simulink model "Simulation_6DOFTesting01"  (R2024a)
settings: Solver=ode4  StartTime=initial_time  StopTime=final_time  FixedStep=timestep  RelTol=1e-3
values from neighbouring files (symbols this model uses):
  aEarth = 0    [CodeTesting_6DOF.m]    (also in Constants_6DOF.m = 6378137; Constants_6DOFTesting.m = 6378137)
  alphaArray = [-30, -25, -20, -15, -10, -5, 0, 5, 10, 15, 20, 25, 30]    [CodeTesting_6DOF.m]    (also in Constants_6DOF.m; Constants_6DOFTesting.m)
  altitudeArray = [0, 1000, 2000, 3000, 4000, 5000, 6000, 7000, 8000, 9000, 10000, 15000, 20000,      25000, 30000, 35000, 40000, 45000, 50000, 55000, 60000]    [CodeTesting_6DOF.m]    (also in Constants_6DOF.m; Constants_6DOFTesting.m)
  bEarth = 0    [CodeTesting_6DOF.m]    (also in Constants_6DOF.m = 6356752.3; Constants_6DOFTesting.m = 6356752.3)
  cD_3DArray = zeros(numAoAs, numMachs, numAltitudes)    [CodeTesting_6DOF.m]    (also in Constants_6DOF.m; Constants_6DOFTesting.m)
  cL_3DArray = zeros(numAoAs, numMachs, numAltitudes)    [CodeTesting_6DOF.m]    (also in Constants_6DOF.m; Constants_6DOFTesting.m)
  densityList = rhoList    [CodeTesting_6DOF.m]    (also in Constants_6DOF.m = usAtmosphere.x_; Constants_6DOFTesting.m = usAtmosphere.x_)
  height0 = 0    [Constants_6DOF.m]    (also in Constants_6DOFTesting.m = 5000)
  heightsList = usAtmosphere.Z    [CodeTesting_6DOF.m]    (also in Constants_6DOF.m; Constants_6DOFTesting.m)
  inertialPitch0 = deg2rad(inertialPitch0)    [Constants_6DOFTesting.m]
  inertialRoll0 = deg2rad(inertialRoll0)    [Constants_6DOFTesting.m]
  inertialYaw0 = deg2rad(inertialYaw0)    [Constants_6DOFTesting.m]
  Ixx = 10    [CodeTesting_6DOF.m]    (also in Constants_6DOF.m; Constants_6DOFTesting.m = 4.88094462)
  Ixz = 10    [CodeTesting_6DOF.m]    (also in Constants_6DOF.m = 1; Constants_6DOFTesting.m = 4.88094462)
  Iyy = 10    [CodeTesting_6DOF.m]    (also in Constants_6DOF.m; Constants_6DOFTesting.m = 4.88094462)
  Izz = 10    [CodeTesting_6DOF.m]    (also in Constants_6DOF.m; Constants_6DOFTesting.m = 4.88094462)
  latitude0 = pi/4    (= 0.785398163397)    [CodeTesting_6DOF.m]    (also in Constants_6DOF.m = deg2rad(latitude0); Constants_6DOFTesting.m = deg2rad(latitude0))
  longitude0 = pi/4    (= 0.785398163397)    [CodeTesting_6DOF.m]    (also in Constants_6DOF.m = deg2rad(longitude0); Constants_6DOFTesting.m = deg2rad(longitude0))
  m0 = 10    [CodeTesting_6DOF.m]    (also in Constants_6DOF.m = 50; Constants_6DOFTesting.m = 14.5939029)
  machArray = [0.5, 1.0, 1.5, 2.0, 2.5, 3.0, 3.5, 4.0, 4.5, 5.0, 5.5, 6.0, 6.5, 7.0, 7.5, 8.0,      8.5, 9.0, 9.5, 10.0]    [CodeTesting_6DOF.m]    (also in Constants_6DOF.m; Constants_6DOFTesting.m)
  omegaEarth = omega_earth    (= 7.2921159e-05)    [CodeTesting_6DOF.m]    (also in Constants_6DOF.m; Constants_6DOFTesting.m)
  p0Body = deg2rad(p0Body)    [Constants_6DOFTesting.m]
  phiBody0 = deg2rad(phiBody0)    [Constants_6DOFTesting.m]
  pitchCharacteristicLength = 0.0    (= 0)    [Constants_6DOFTesting.m]
  psiBody0 = deg2rad(psiBody0)    [Constants_6DOFTesting.m]
  q0Body = deg2rad(q0Body)    [Constants_6DOFTesting.m]
  r0Body = deg2rad(r0Body)    [Constants_6DOFTesting.m]
  rEarth = r_earth    (= 6371008.8)    [CodeTesting_6DOF.m]    (also in Constants_6DOF.m; Constants_6DOFTesting.m)
  rollCharacteristicLength = 0.0    (= 0)    [Constants_6DOFTesting.m]
  temperatureList = usAtmosphere.T    [CodeTesting_6DOF.m]    (also in Constants_6DOF.m; Constants_6DOFTesting.m)
  thetaBody0 = deg2rad(thetaBody0)    [Constants_6DOFTesting.m]
  u0Body = 304.8    [Constants_6DOFTesting.m]
  v0Body = 0    [Constants_6DOFTesting.m]
  w0Body = -1 * w0Body    (= 0)    [Constants_6DOFTesting.m]
  wingArea = 0    [CodeTesting_6DOF.m]    (also in Constants_6DOF.m = 50; Constants_6DOFTesting.m = 0.09290304)
  yawCharacteristicLength = 0.0    (= 0)    [Constants_6DOFTesting.m]
undefined symbols (not defined in the file or in its folder): inertialX0, inertialY0, inertialZ0
libraries: simulink_extras x28
(part 2 of 2)

== matlab function Simulation_6DOFTesting01/Coordinate Transformations/ecef2ned ==
  data: positionECEF input; y output; latitude input; longitude input
function y = fcn(positionECEF, latitude, longitude)

rotationMatrix = [-sin(latitude) * cos(longitude) -sin(latitude) * sin(longitude) cos(latitude); -sin(longitude) cos(longitude) 0; -cos(latitude) * cos(longitude) -cos(latitude) * sin(longitude) sin(latitude)];

nedPosition = rotationMatrix * positionECEF;

y = nedPosition;

== matlab function Simulation_6DOFTesting01/Control Surfaces/bankAngle ==
  data: t input; y output
function y = fcn(t)

bankAngle = 0;

y = bankAngle;

== matlab function Simulation_6DOFTesting01/Forces, Moments & their Coefficients/rollCoeff ==
  data: rollSurfaceDeflection input; y output
function y = fcn(rollSurfaceDeflection)

staticRollCoeff = rollSurfaceDeflection;
dynamicRollCoeff = 0.0;

rollCoeff = staticRollCoeff + dynamicRollCoeff;

y = rollCoeff;

== matlab function Simulation_6DOFTesting01/Forces, Moments & their Coefficients/pitchCoeff ==
  data: pitchSurfaceDeflection input; y output
function y = fcn(pitchSurfaceDeflection)

staticPitchCoeff = pitchSurfaceDeflection;
dynamicPitchCoeff = 0.0;

pitchCoeff = staticPitchCoeff + dynamicPitchCoeff;

y = pitchCoeff;

== matlab function Simulation_6DOFTesting01/Forces, Moments & their Coefficients/yawCoeff ==
  data: yawSurfaceDeflection input; y output
function y = fcn(yawSurfaceDeflection)

staticYawCoeff = yawSurfaceDeflection;
dynamicYawCoeff = 0.0;

yawCoeff = staticYawCoeff + dynamicYawCoeff;

y = yawCoeff;

== matlab function Simulation_6DOFTesting01/Constants & Aircraft Parameters/thrustBurnRate ==
  data: t input; y output
function y = fcn(t)

thrustBurnRate = 0;

y = thrustBurnRate;

== matlab function Simulation_6DOFTesting01/Forces, Moments & their Coefficients/Fx ==
  data: thrustX input; y output; gravityX input; dragX input; coriolisX input
function y = fcn(thrustX, gravityX, dragX, coriolisX)

xForce = thrustX + gravityX + coriolisX - dragX;

y = xForce;

== matlab function Simulation_6DOFTesting01/Forces, Moments & their Coefficients/Fy ==
  data: thrustY input; y output; gravityY input; coriolisY input
function y = fcn(thrustY, gravityY, coriolisY)

yForce = thrustY + gravityY + coriolisY;

y = yForce;

== matlab function Simulation_6DOFTesting01/Forces, Moments & their Coefficients/Fz ==
  data: thrustZ input; y output; gravityZ input; liftZ input; coriolisZ input
function y = fcn(thrustZ, gravityZ, liftZ, coriolisZ)

zForce = thrustZ + gravityZ + coriolisZ - liftZ;

y = zForce;

== matlab function Simulation_6DOFTesting01/Forces, Moments & their Coefficients/MATLAB Function ==
  data: thrustX input; y output; thrustY input; thrustZ input
function y = fcn(thrustX, thrustY, thrustZ)

thrustMagnitude = sqrt(thrustX^2 + thrustY^2 + thrustZ^2);

y = thrustMagnitude;

== matlab function Simulation_6DOFTesting01/Coordinate Transformations/Subsystem/velocity ==
  data: u input; y output; v input; w input
function y = fcn(u, v, w)

velocity = sqrt(u^2 + v^2 + w^2);

y = velocity;

== matlab function Simulation_6DOFTesting01/Forces, Moments & their Coefficients/MATLAB Function1 ==
  data: forceVector input; y output; AoA input; sideslip input
function y = fcn(forceVector, AoA, sideslip)

rotationMatrix = [cos(AoA) * cos(sideslip) -cos(AoA) * sin(sideslip) -sin(AoA); sin(sideslip) cos(sideslip) 0; sin(AoA) * cos(sideslip) -sin(AoA) * sin(sideslip) cos(AoA)];

rotatedForceVector = rotationMatrix * forceVector;

y = rotatedForceVector;

== matlab function Simulation_6DOFTesting01/Forces, Moments & their Coefficients/MATLAB Function2 ==
  data: m input; g input; psi input; theta input; phi input; AoA input; y output; sideslip input
function y = fcn(m, g, psi, theta, phi, AoA, sideslip)

inertialGravity = [0; 0; m * g];

x0 = cos(psi);
x1 = cos(theta);
x2 = sin(psi);
x3 = sin(theta);
x4 = cos(phi);
x5 = x2*x4;
x6 = sin(phi);
x7 = x0*x6;
x8 = x0*x4;
x9 = x2*x6;

rotationMatrixBI = [x0 * x1 x3 * x7 - x5 x3 * x8 + x9; x1 * x2 x3 * x9 + x8 x3 * x5 - x7; -x3 x1 * x6 x1 * x4];

rotationBI = inv(rotationMatrixBI);
rotationWB = [cos(AoA) * cos(sideslip) -cos(AoA) * sin(sideslip) -sin(AoA); sin(sideslip) cos(sideslip) 0; sin(AoA) * cos(sideslip) -sin(AoA) * sin(sideslip) cos(AoA)];

bodyGravity = rotationBI * inertialGravity;
windGravity = rotationWB * bodyGravity;

y = windGravity;

== matlab function Simulation_6DOFTesting01/Equations of Motion/Subsystem2/MATLAB Function1 ==
  data: r input; y output; q input; phi input
function y = fcn(r, q, phi)

y = q * cos(phi) - r * sin(phi);

== matlab function Simulation_6DOFTesting01/Equations of Motion/Subsystem2/MATLAB Function2 ==
  data: r input; y output; q input; phi input; theta input
function y = fcn(r, q, phi, theta)

y = q * sin(phi) * sec(theta) + r * cos(phi) * sec(theta);

== matlab function Simulation_6DOFTesting01/Control Surfaces/sideslipAngle ==
  data: t input; y output
function y = fcn(t)

sideslipAngle = 0;

y = sideslipAngle;

== matlab function Simulation_6DOFTesting01/Equations of Motion/Subsystem2/MATLAB Function3 ==
  data: omegaEarth input; y output; latitude input; longitude input; positionNED input
function y = fcn(omegaEarth, latitude, longitude, positionNED)

omegaEarth = [0; 0; omegaEarth];

lat = latitude;
long = longitude;

row1 = [-cos(long) * sin(lat) -sin(long) -cos(lat) * cos(long)];
row2 = [-sin(lat) * sin(long) cos(long) -cos(lat) * sin(long)];
row3 = [cos(lat) 0 -sin(lat)];

rotationMatrix = inv([row1; row2; row3]);
velocityNEDFrame = rotationMatrix * omegaEarth;
positionNED = positionNED;

velNEDX = velocityNEDFrame(1);
velNEDY = velocityNEDFrame(2);
velNEDZ = velocityNEDFrame(3);

posNEDX = positionNED(1);
posNEDY = positionNED(2);
posNEDZ = positionNED(3);

velRotEarthX = velNEDY * posNEDZ - velNEDZ * posNEDY;
velRotEarthY = velNEDZ * posNEDX - velNEDX * posNEDZ;
velRotEarthZ = velNEDX * posNEDY - velNEDY * posNEDX;

velocityRotatingEarth = [velRotEarthX; velRotEarthY; velRotEarthZ];

y = velocityRotatingEarth;

== matlab function Simulation_6DOFTesting01/Equations of Motion/Subsystem2/MATLAB Function4 ==
  data: velocityRotatingEarth input; y output
function y = fcn(velocityRotatingEarth)

magnitudeRotatingEarth = norm(velocityRotatingEarth);

y = magnitudeRotatingEarth;

== matlab function Simulation_6DOFTesting01/Coordinate Transformations/MATLAB Function ==
  data: positionNED input; y output; latitude input; longitude input
function y = fcn(positionNED, latitude, longitude)

rotationY = roty(pi/2 + latitude);
rotationZ = rotz(-1 * longitude);

rotationMatrix = rotationZ * rotationY;

cartesianECEF = rotationMatrix * positionNED;

y = cartesianECEF;

== matlab function Simulation_6DOFTesting01/Coordinate Transformations/Polar ECEF - lat, long, height/MATLAB Function ==
  data: a input; y output; b input; xECEF input; yECEF input; latitude input; height0 input
function y = fcn(a, b, xECEF, yECEF, latitude, height0)

e = sqrt(1 - b^2/a^2);
p = sqrt(xECEF^2 + yECEF^2);

N = a / sqrt(1 - e^2 * sin(latitude)^2);
alt = p / cos(latitude) - (N + height0);


y = alt;

== matlab function Simulation_6DOFTesting01/Forces, Moments & their Coefficients/Coriolis Force ==
  data: m input; y output; omegaEarth input; latitude input; longitude input; vNEDX input; vNEDY input; vNEDZ input
function y = fcn(m, omegaEarth, latitude, longitude, vNEDX, vNEDY, vNEDZ)

lat = latitude;
long = longitude;

row1 = [-cos(long) * sin(lat) -sin(long) -cos(lat) * cos(long)];
row2 = [-sin(lat) * sin(long) cos(long) -cos(lat) * sin(long)];
row3 = [cos(lat) 0 -sin(lat)];

rotationMatrix = inv([row1; row2; row3]);
omegaNED = rotationMatrix * [0; 0; omegaEarth];

omegNEDX = omegaNED(1);
omegNEDY = omegaNED(2);
omegNEDZ = omegaNED(3);

coriolisX = -2 * m * (omegNEDY * vNEDZ - omegNEDZ * vNEDY);
coriolisY = -2 * m * (omegNEDZ * vNEDX - omegNEDX * vNEDZ);
coriolisZ = -2 * m * (omegNEDX * vNEDY - omegNEDY * vNEDX);

coriolisX = 0;
coriolisY = 0;
coriolisZ = 0;

coriolisForce = [coriolisX; coriolisY; coriolisZ];

y = coriolisForce;

== matlab function Simulation_6DOFTesting01/Control Surfaces/AoA ==
  data: t input; y output
function y = fcn(t)

AoA = 0;

y = AoA;

== matlab function Simulation_6DOFTesting01/Equations of Motion/Subsystem1/MATLAB Function2 ==
  data: angleVector input; y output; phi input; theta input; psi input
function y = fcn(angleVector, phi, theta, psi)

x0 = cos(psi);
x1 = cos(theta);
x2 = sin(psi);
x3 = sin(theta);
x4 = cos(phi);
x5 = x2*x4;
x6 = sin(phi);
x7 = x0*x6;
x8 = x0*x4;
x9 = x2*x6;

rotationMatrixIB = [x0 * x1 x3 * x7 - x5 x3 * x8 + x9; x1 * x2 x3 * x9 + x8 x3 * x5 - x7; -x3 x1 * x6 x1 * x4];

angleVectorNED = rotationMatrixIB * angleVector;

y = angleVectorNED;

== matlab function Simulation_6DOFTesting01/Coordinate Transformations/Cartesian ECEF - x, y, z/MATLAB Function4 ==
  data: positionECEF input; y output
function y = fcn(positionECEF)

rEarth = 6371.0088 * 10^3;

height = norm(positionECEF) - rEarth;

y = height;

== matlab function Simulation_6DOFTesting01/Equations of Motion/Subsystem1/MATLAB Function3 ==
  data: psi input; y output; theta input; phi input
function y = fcn(psi, theta, phi)

initialAngleVector = [phi; theta; psi];

x0 = cos(psi);
x1 = cos(theta);
x2 = sin(psi);
x3 = sin(theta);
x4 = cos(phi);
x5 = x2*x4;
x6 = sin(phi);
x7 = x0*x6;
x8 = x0*x4;
x9 = x2*x6;

rotationMatrixIB = [x0 * x1 x3 * x7 - x5 x3 * x8 + x9; x1 * x2 x3 * x9 + x8 x3 * x5 - x7; -x3 x1 * x6 x1 * x4];

eulerAngles = rotationMatrixIB * initialAngleVector;

y = eulerAngles;

== matlab function Simulation_6DOFTesting01/Coordinate Transformations/Cartesian ECEF - x, y, z/MATLAB Function ==
  data: u input; y output
function y = fcn(u)

y = norm(u);

== matlab function Simulation_6DOFTesting01/Coordinate Transformations/Polar ECEF - lat, long, height/MATLAB Function4 ==
  data: u input; y output
function y = fcn(u)

y = norm(u);

== matlab function Simulation_6DOFTesting01/Coordinate Transformations/Polar ECEF - lat, long, height/MATLAB Function5 ==
  data: latitude input; longitude input; positionNED input; y output; latitude0 input; longitude0 input; height0 input; a input; b input; t input
function y = fcn( latitude, longitude, positionNED, latitude0, longitude0, height0, a, b, t)

rEarth = 6371.0088 * 10^3; 

long = longitude;
lat = latitude;

row1 = [-cos(long) * sin(lat) -sin(long) -cos(lat) * cos(long)];
row2 = [-sin(lat) * sin(long) cos(long) -cos(lat) * sin(long)];
row3 = [cos(lat) 0 -sin(lat)];

rotationMatrix = [row1; row2; row3];

positionNED(3) = positionNED(3);

e = sqrt(1 - b^2/a^2);
N = a * (1 - e^2 * sin(latitude0)^2)^(-1/2);

initialECEFX = (height0 + N) * cos(latitude0) * cos(longitude0);
initialECEFY = (height0 + N) * cos(latitude0) * sin(longitude0);
initialECEFZ = (height0 + N * (1 - e^2)) * sin(latitude0);

initialECEFPosition = [initialECEFX; initialECEFY; initialECEFZ];


positionECEF = rotationMatrix * positionNED + initialECEFPosition;

y = positionECEF;

== matlab function Simulation_6DOFTesting01/Coordinate Transformations/Polar ECEF - lat, long, height/MATLAB Function6 ==
  data: t input; y output; latitude0 input; xECEF input; yECEF input; zECEF input; a input; b input
function y = fcn(t, latitude0, xECEF, yECEF, zECEF, a, b)

e = sqrt(1 - b^2/a^2);
e2 = sqrt(a^2/b^2 - 1);
p = sqrt(xECEF^2 + yECEF^2);

theta = atan2(zECEF * a, p * b);
lat = atan2(zECEF + e2^2 * b * sin(theta)^3, p - e^2 * a * cos(theta)^3);

if t == 0
    latitude = latitude0;
else
    latitude = lat;
end

y = latitude;

== matlab function Simulation_6DOFTesting01/Control Surfaces/rollSurfaceDeflection ==
  data: t input; y output
function y = fcn(t)

rollSurfaceDeflection = 0.0;

y = rollSurfaceDeflection;

== matlab function Simulation_6DOFTesting01/Coordinate Transformations/Polar ECEF - lat, long, height/MATLAB Function7 ==
  data: t input; y output; longitude0 input; xECEF input; yECEF input
function y = fcn(t, longitude0, xECEF, yECEF)

long = atan2(yECEF, xECEF);

if t == 0
    long = longitude0;
else
    long = atan2(yECEF, xECEF);
end

longitude = long;

y = longitude;

== matlab function Simulation_6DOFTesting01/Equations of Motion/Subsystem1/MATLAB Function4 ==
  data: angleRateVector input; y output; phi input; theta input; psi input
function y = fcn(angleRateVector, phi, theta, psi)

x0 = cos(psi);
x1 = cos(theta);
x2 = sin(psi);
x3 = sin(theta);
x4 = cos(phi);
x5 = x2*x4;
x6 = sin(phi);
x7 = x0*x6;
x8 = x0*x4;
x9 = x2*x6;

rotationMatrixIB = [x0 * x1 x3 * x7 - x5 x3 * x8 + x9; x1 * x2 x3 * x9 + x8 x3 * x5 - x7; -x3 x1 * x6 x1 * x4];

angleRateVectorNED = rotationMatrixIB * angleRateVector;

y = angleRateVectorNED;

== matlab function Simulation_6DOFTesting01/Forces, Moments & their Coefficients/LiftZ ==
  data: rho input; y output; cl input; A input; v input
function y = fcn(rho, cl, A, v)

Lift =  0.5 * rho * v^2 * A * cl;
Lift = 0;

y = Lift;

== matlab function Simulation_6DOFTesting01/Forces, Moments & their Coefficients/DragX ==
  data: rho input; y output; v input; cd input; A input
function y = fcn(rho, v, cd, A)

cd = 0.1;
Drag = 0.5 * rho * v^2 * A * cd;

y = Drag;

== matlab function Simulation_6DOFTesting01/Atmospheric Conditions/g ==
  data: y output; r input
function y = fcn(r)

mu_earth = 3.986004418 * 10^14;
rE = 6378140;

y = mu_earth / (rE + r)^2;

== matlab function Simulation_6DOFTesting01/Atmospheric Conditions/rho ==
  data: rhoList input; hList input; r input; y output
function y = fcn(rhoList, hList, r)

r = r / 10^3;

if r >= 0
    density = interp1(hList, rhoList, r);
else
    density = 0;
end


y = density;
